simulink model "physical_architecture"  (R2019b)
settings: Solver=VariableStepAuto  StartTime=0.0  StopTime=10.0  RelTol=1e-3
settings Model: Creator=nicol  LastModifiedBy=nicol

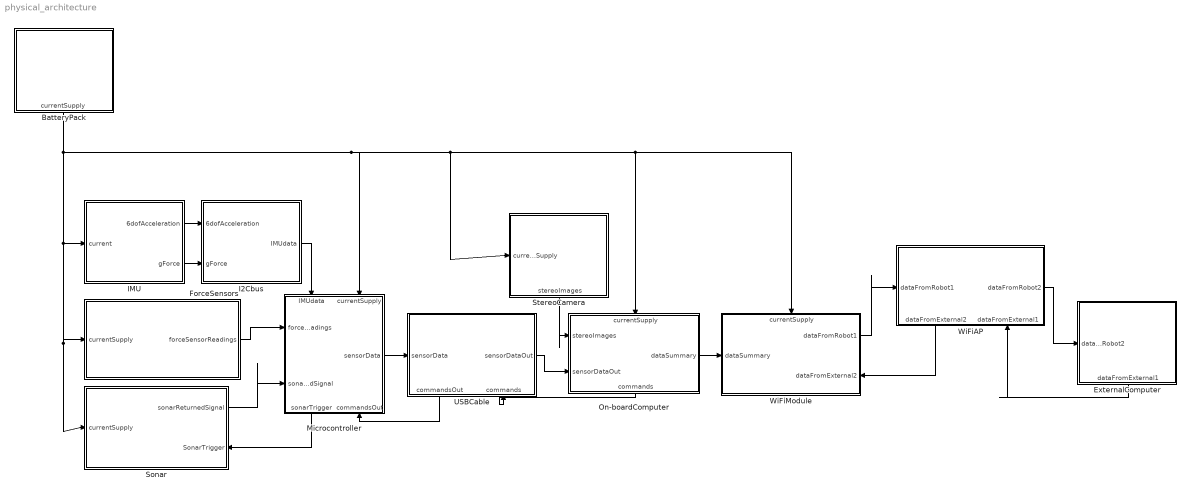
== system physical_architecture ==
  BatteryPack : Subsystem
      settings: PortSchema="{\"entries\":[{\"content\":{\"headerSize\":26,\"margin\":15,\"minimumSpacing\":25,\"sides\":[{\"content\":{\"connectorIds\":[]},\"type\":\"ConnectorPlacement.EquallySpacedRectSide\",\"uuid\":\"1a5b96a6-6b68-4a44-94ba-f4f30127e72c\"},{\"content\":{\"connectorIds\":[],\"side\":\"RIGHT\"},\"type\":\"ConnectorPlacement.EquallySpacedRectSide\",\"uuid\":\"6795999a-37c2-4f74-9b2a-5ff47da3b2b8\"},{\"content\":{\"connectorIds\":[],\"side\":\"TOP\"},\"type\":\"ConnectorPlacement.EquallySpacedRectSide\",\"uuid\":\"71a167ad-2262-404f-8290-656c4c9ef881\"},{\"content\":{\"connectorIds\":[\"Out1\"],\"side\":\"BOTTOM\"},\"type\":\"ConnectorPlacement.EquallySpacedRectSide\",\"uuid\":\"0e7f1ae4-2808-47ff-a788-11b0bf7ea7a5\"}]},\"type\":\"ConnectorPlacement.EquallySpacedConnector\",\"uuid\":\"f8e426a6-4f1d-49ba-8aa9-835f0600076a\"}],\"packageUris\":[\"http://schema.mathworks.com/mf0/Connector/19700101\"],\"version\":\"1.0\"}"
  ExternalComputer : Subsystem
      settings: PortSchema="{\"entries\":[{\"content\":{\"headerSize\":26,\"margin\":15,\"minimumSpacing\":25,\"sides\":[{\"content\":{\"connectorIds\":[\"In1\"]},\"type\":\"ConnectorPlacement.EquallySpacedRectSide\",\"uuid\":\"1a5b96a6-6b68-4a44-94ba-f4f30127e72c\"},{\"content\":{\"connectorIds\":[],\"side\":\"RIGHT\"},\"type\":\"ConnectorPlacement.EquallySpacedRectSide\",\"uuid\":\"6795999a-37c2-4f74-9b2a-5ff47da3b2b8\"},{\"content\":{\"connectorIds\":[],\"side\":\"TOP\"},\"type\":\"ConnectorPlacement.EquallySpacedRectSide\",\"uuid\":\"71a167ad-2262-404f-8290-656c4c9ef881\"},{\"content\":{\"connectorIds\":[\"Out1\"],\"side\":\"BOTTOM\"},\"type\":\"ConnectorPlacement.EquallySpacedRectSide\",\"uuid\":\"2cc7744c-30d7-486d-8de8-8132ed659702\"}]},\"type\":\"ConnectorPlacement.EquallySpacedConnector\",\"uuid\":\"f8e426a6-4f1d-49ba-8aa9-835f0600076a\"}],\"packageUris\":[\"http://schema.mathworks.com/mf0/Connector/19700101\"],\"version\":\"1.0\"}"
  ForceSensors : Subsystem
      settings: PortSchema="{\"entries\":[{\"content\":{\"headerSize\":26,\"margin\":15,\"minimumSpacing\":25,\"sides\":[{\"content\":{\"connectorIds\":[\"In1\"]},\"type\":\"ConnectorPlacement.EquallySpacedRectSide\",\"uuid\":\"1a5b96a6-6b68-4a44-94ba-f4f30127e72c\"},{\"content\":{\"connectorIds\":[\"Out1\"],\"side\":\"RIGHT\"},\"type\":\"ConnectorPlacement.EquallySpacedRectSide\",\"uuid\":\"6795999a-37c2-4f74-9b2a-5ff47da3b2b8\"},{\"content\":{\"connectorIds\":[],\"side\":\"TOP\"},\"type\":\"ConnectorPlacement.EquallySpacedRectSide\",\"uuid\":\"71a167ad-2262-404f-8290-656c4c9ef881\"}]},\"type\":\"ConnectorPlacement.EquallySpacedConnector\",\"uuid\":\"f8e426a6-4f1d-49ba-8aa9-835f0600076a\"}],\"packageUris\":[\"http://schema.mathworks.com/mf0/Connector/19700101\"],\"version\":\"1.0\"}"
  I2Cbus : Subsystem
      settings: PortSchema="{\"entries\":[{\"content\":{\"headerSize\":26,\"margin\":15,\"minimumSpacing\":25,\"sides\":[{\"content\":{\"connectorIds\":[\"In1\",\"In2\"]},\"type\":\"ConnectorPlacement.EquallySpacedRectSide\",\"uuid\":\"1a5b96a6-6b68-4a44-94ba-f4f30127e72c\"},{\"content\":{\"connectorIds\":[\"Out1\"],\"side\":\"RIGHT\"},\"type\":\"ConnectorPlacement.EquallySpacedRectSide\",\"uuid\":\"6795999a-37c2-4f74-9b2a-5ff47da3b2b8\"},{\"content\":{\"connectorIds\":[],\"side\":\"TOP\"},\"type\":\"ConnectorPlacement.EquallySpacedRectSide\",\"uuid\":\"71a167ad-2262-404f-8290-656c4c9ef881\"}]},\"type\":\"ConnectorPlacement.EquallySpacedConnector\",\"uuid\":\"f8e426a6-4f1d-49ba-8aa9-835f0600076a\"}],\"packageUris\":[\"http://schema.mathworks.com/mf0/Connector/19700101\"],\"version\":\"1.0\"}"
  IMU : Subsystem
      settings: PortSchema="{\"entries\":[{\"content\":{\"headerSize\":26,\"margin\":15,\"minimumSpacing\":25,\"sides\":[{\"content\":{\"connectorIds\":[\"In1\"]},\"type\":\"ConnectorPlacement.EquallySpacedRectSide\",\"uuid\":\"1a5b96a6-6b68-4a44-94ba-f4f30127e72c\"},{\"content\":{\"connectorIds\":[\"Out1\",\"Out2\"],\"side\":\"RIGHT\"},\"type\":\"ConnectorPlacement.EquallySpacedRectSide\",\"uuid\":\"6795999a-37c2-4f74-9b2a-5ff47da3b2b8\"},{\"content\":{\"connectorIds\":[],\"side\":\"TOP\"},\"type\":\"ConnectorPlacement.EquallySpacedRectSide\",\"uuid\":\"71a167ad-2262-404f-8290-656c4c9ef881\"}]},\"type\":\"ConnectorPlacement.EquallySpacedConnector\",\"uuid\":\"f8e426a6-4f1d-49ba-8aa9-835f0600076a\"}],\"packageUris\":[\"http://schema.mathworks.com/mf0/Connector/19700101\"],\"version\":\"1.0\"}"
  Microcontroller : Subsystem
      settings: PortSchema="{\"entries\":[{\"content\":{\"headerSize\":26,\"margin\":15,\"minimumSpacing\":25,\"sides\":[{\"content\":{\"connectorIds\":[\"In2\",\"In4\"]},\"type\":\"ConnectorPlacement.EquallySpacedRectSide\",\"uuid\":\"1a5b96a6-6b68-4a44-94ba-f4f30127e72c\"},{\"content\":{\"connectorIds\":[\"Out1\"],\"side\":\"RIGHT\"},\"type\":\"ConnectorPlacement.EquallySpacedRectSide\",\"uuid\":\"6795999a-37c2-4f74-9b2a-5ff47da3b2b8\"},{\"content\":{\"connectorIds\":[\"In5\",\"In3\"],\"side\":\"TOP\"},\"type\":\"ConnectorPlacement.EquallySpacedRectSide\",\"uuid\":\"71a167ad-2262-404f-8290-656c4c9ef881\"},{\"content\":{\"connectorIds\":[\"Out2\",\"In1\"],\"side\":\"BOTTOM\"},\"type\":\"ConnectorPlacement.EquallySpacedRectSide\",\"uuid\":\"845b4600-6435-40f5-ac3b-dfa55e6d602e\"}]},\"type\":\"ConnectorPlacement.EquallySpacedConnector\",\"uuid\":\"f8e426a6-4f1d-49ba-8aa9-835f0600076a\"}],\"packageUris\":[\"http://schema.mathworks.com/mf0/Connector/19700101\"],\"version\":\"1.0\"}"
  On-boardComputer : Subsystem
      settings: PortSchema="{\"entries\":[{\"content\":{\"headerSize\":26,\"margin\":15,\"minimumSpacing\":25,\"sides\":[{\"content\":{\"connectorIds\":[\"In2\",\"In3\"]},\"type\":\"ConnectorPlacement.EquallySpacedRectSide\",\"uuid\":\"1a5b96a6-6b68-4a44-94ba-f4f30127e72c\"},{\"content\":{\"connectorIds\":[\"Out1\"],\"side\":\"RIGHT\"},\"type\":\"ConnectorPlacement.EquallySpacedRectSide\",\"uuid\":\"6795999a-37c2-4f74-9b2a-5ff47da3b2b8\"},{\"content\":{\"connectorIds\":[\"In1\"],\"side\":\"TOP\"},\"type\":\"ConnectorPlacement.EquallySpacedRectSide\",\"uuid\":\"71a167ad-2262-404f-8290-656c4c9ef881\"},{\"content\":{\"connectorIds\":[\"Out2\"],\"side\":\"BOTTOM\"},\"type\":\"ConnectorPlacement.EquallySpacedRectSide\",\"uuid\":\"e904cf2f-4a71-419b-a2b8-63e25171dc86\"}]},\"type\":\"ConnectorPlacement.EquallySpacedConnector\",\"uuid\":\"f8e426a6-4f1d-49ba-8aa9-835f0600076a\"}],\"packageUris\":[\"http://schema.mathworks.com/mf0/Connector/19700101\"],\"version\":\"1.0\"}"
  Sonar : Subsystem
      settings: PortSchema="{\"entries\":[{\"content\":{\"headerSize\":26,\"margin\":15,\"minimumSpacing\":25,\"sides\":[{\"content\":{\"connectorIds\":[\"In1\"]},\"type\":\"ConnectorPlacement.EquallySpacedRectSide\",\"uuid\":\"1a5b96a6-6b68-4a44-94ba-f4f30127e72c\"},{\"content\":{\"connectorIds\":[\"Out1\",\"In2\"],\"side\":\"RIGHT\"},\"type\":\"ConnectorPlacement.EquallySpacedRectSide\",\"uuid\":\"6795999a-37c2-4f74-9b2a-5ff47da3b2b8\"},{\"content\":{\"connectorIds\":[],\"side\":\"TOP\"},\"type\":\"ConnectorPlacement.EquallySpacedRectSide\",\"uuid\":\"71a167ad-2262-404f-8290-656c4c9ef881\"}]},\"type\":\"ConnectorPlacement.EquallySpacedConnector\",\"uuid\":\"f8e426a6-4f1d-49ba-8aa9-835f0600076a\"}],\"packageUris\":[\"http://schema.mathworks.com/mf0/Connector/19700101\"],\"version\":\"1.0\"}"
  StereoCamera : Subsystem
      settings: PortSchema="{\"entries\":[{\"content\":{\"headerSize\":26,\"margin\":15,\"minimumSpacing\":25,\"sides\":[{\"content\":{\"connectorIds\":[\"In1\"]},\"type\":\"ConnectorPlacement.EquallySpacedRectSide\",\"uuid\":\"1a5b96a6-6b68-4a44-94ba-f4f30127e72c\"},{\"content\":{\"connectorIds\":[],\"side\":\"RIGHT\"},\"type\":\"ConnectorPlacement.EquallySpacedRectSide\",\"uuid\":\"6795999a-37c2-4f74-9b2a-5ff47da3b2b8\"},{\"content\":{\"connectorIds\":[],\"side\":\"TOP\"},\"type\":\"ConnectorPlacement.EquallySpacedRectSide\",\"uuid\":\"71a167ad-2262-404f-8290-656c4c9ef881\"},{\"content\":{\"connectorIds\":[\"Out1\"],\"side\":\"BOTTOM\"},\"type\":\"ConnectorPlacement.EquallySpacedRectSide\",\"uuid\":\"983849b7-be9a-4e5c-b816-a95c1f7f6796\"}]},\"type\":\"ConnectorPlacement.EquallySpacedConnector\",\"uuid\":\"f8e426a6-4f1d-49ba-8aa9-835f0600076a\"}],\"packageUris\":[\"http://schema.mathworks.com/mf0/Connector/19700101\"],\"version\":\"1.0\"}"
  USBCable : Subsystem
      settings: PortSchema="{\"entries\":[{\"content\":{\"headerSize\":26,\"margin\":15,\"minimumSpacing\":25,\"sides\":[{\"content\":{\"connectorIds\":[\"In2\"]},\"type\":\"ConnectorPlacement.EquallySpacedRectSide\",\"uuid\":\"1a5b96a6-6b68-4a44-94ba-f4f30127e72c\"},{\"content\":{\"connectorIds\":[\"Out2\"],\"side\":\"RIGHT\"},\"type\":\"ConnectorPlacement.EquallySpacedRectSide\",\"uuid\":\"6795999a-37c2-4f74-9b2a-5ff47da3b2b8\"},{\"content\":{\"connectorIds\":[],\"side\":\"TOP\"},\"type\":\"ConnectorPlacement.EquallySpacedRectSide\",\"uuid\":\"71a167ad-2262-404f-8290-656c4c9ef881\"},{\"content\":{\"connectorIds\":[\"Out1\",\"In1\"],\"side\":\"BOTTOM\"},\"type\":\"ConnectorPlacement.EquallySpacedRectSide\",\"uuid\":\"96aedcb9-6a36-4cb0-8a83-77dcedd4fe91\"}]},\"type\":\"ConnectorPlacement.EquallySpacedConnector\",\"uuid\":\"f8e426a6-4f1d-49ba-8aa9-835f0600076a\"}],\"packageUris\":[\"http://schema.mathworks.com/mf0/Connector/19700101\"],\"version\":\"1.0\"}"
  WiFiAP : Subsystem
      settings: PortSchema="{\"entries\":[{\"content\":{\"headerSize\":26,\"margin\":15,\"minimumSpacing\":25,\"sides\":[{\"content\":{\"connectorIds\":[\"In2\"]},\"type\":\"ConnectorPlacement.EquallySpacedRectSide\",\"uuid\":\"1a5b96a6-6b68-4a44-94ba-f4f30127e72c\"},{\"content\":{\"connectorIds\":[\"Out2\"],\"side\":\"RIGHT\"},\"type\":\"ConnectorPlacement.EquallySpacedRectSide\",\"uuid\":\"6795999a-37c2-4f74-9b2a-5ff47da3b2b8\"},{\"content\":{\"connectorIds\":[],\"side\":\"TOP\"},\"type\":\"ConnectorPlacement.EquallySpacedRectSide\",\"uuid\":\"71a167ad-2262-404f-8290-656c4c9ef881\"},{\"content\":{\"connectorIds\":[\"Out1\",\"In1\"],\"side\":\"BOTTOM\"},\"type\":\"ConnectorPlacement.EquallySpacedRectSide\",\"uuid\":\"aacabda8-2325-475d-956c-e2fb6a2fac11\"}]},\"type\":\"ConnectorPlacement.EquallySpacedConnector\",\"uuid\":\"f8e426a6-4f1d-49ba-8aa9-835f0600076a\"}],\"packageUris\":[\"http://schema.mathworks.com/mf0/Connector/19700101\"],\"version\":\"1.0\"}"
  WiFiModule : Subsystem
      settings: PortSchema="{\"entries\":[{\"content\":{\"headerSize\":26,\"margin\":15,\"minimumSpacing\":25,\"sides\":[{\"content\":{\"connectorIds\":[\"In3\"]},\"type\":\"ConnectorPlacement.EquallySpacedRectSide\",\"uuid\":\"1a5b96a6-6b68-4a44-94ba-f4f30127e72c\"},{\"content\":{\"connectorIds\":[\"Out1\",\"In2\"],\"side\":\"RIGHT\"},\"type\":\"ConnectorPlacement.EquallySpacedRectSide\",\"uuid\":\"6795999a-37c2-4f74-9b2a-5ff47da3b2b8\"},{\"content\":{\"connectorIds\":[\"In1\"],\"side\":\"TOP\"},\"type\":\"ConnectorPlacement.EquallySpacedRectSide\",\"uuid\":\"71a167ad-2262-404f-8290-656c4c9ef881\"}]},\"type\":\"ConnectorPlacement.EquallySpacedConnector\",\"uuid\":\"f8e426a6-4f1d-49ba-8aa9-835f0600076a\"}],\"packageUris\":[\"http://schema.mathworks.com/mf0/Connector/19700101\"],\"version\":\"1.0\"}"
  wires:
  IMU/1(6dofAcceleration) -> I2Cbus/1(6dofAcceleration)
  IMU/2(gForce) -> I2Cbus/2(gForce)
  I2Cbus/1(IMUdata) -> Microcontroller/5(IMUdata)
  ForceSensors/1(forceSensorReadings) -> Microcontroller/2(forceSensorReadings)
  Sonar/1(sonarReturnedSignal) -> Microcontroller/4(sonarReturnedSignal)
  Microcontroller/2(sonarTrigger) -> Sonar/2(SonarTrigger)
  Microcontroller/1(sensorData) -> USBCable/2(sensorData)
  USBCable/2(sensorDataOut) -> On-boardComputer/3(sensorDataOut)
  On-boardComputer/2(commands) -> USBCable/1(commands)
  On-boardComputer/1(dataSummary) -> WiFiModule/3(dataSummary)
  WiFiModule/1(dataFromRobot1) -> WiFiAP/2(dataFromRobot1)
  WiFiAP/2(dataFromRobot2) -> ExternalComputer/1(dataFromRobot2)
  ExternalComputer/1(dataFromExternal1) -> WiFiAP/1(dataFromExternal1)
  WiFiAP/1(dataFromExternal2) -> WiFiModule/2(dataFromExternal2)
  StereoCamera/1(stereoImages) -> On-boardComputer/2(stereoImages)
  BatteryPack/1(currentSupply) -> StereoCamera/1(currentSupply), WiFiModule/1(currentSupply), On-boardComputer/1(currentSupply), Microcontroller/3(currentSupply), Sonar/1(currentSupply), ForceSensors/1(currentSupply), IMU/1(current)
  USBCable/1(commandsOut) -> Microcontroller/1(commandsOut)

== system physical_architecture/BatteryPack ==
  Bus Element Out1 : Outport  PortName=currentSupply

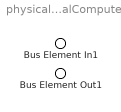
== system physical_architecture/ExternalComputer ==
  Bus Element In1 : Inport  PortName=dataFromRobot2
  Bus Element Out1 : Outport  PortName=dataFromExternal1

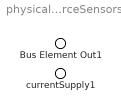
== system physical_architecture/ForceSensors ==
  currentSupply1 : Inport  PortName=currentSupply
  Bus Element Out1 : Outport  PortName=forceSensorReadings

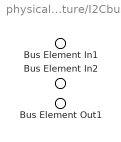
== system physical_architecture/I2Cbus ==
  Bus Element In1 : Inport  PortName=6dofAcceleration
  Bus Element In2 : Inport  Port=2  PortName=gForce
  Bus Element Out1 : Outport  PortName=IMUdata

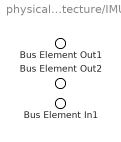
== system physical_architecture/IMU ==
  Bus Element In1 : Inport  PortName=current
  Bus Element Out1 : Outport  PortName=6dofAcceleration
  Bus Element Out2 : Outport  Port=2  PortName=gForce

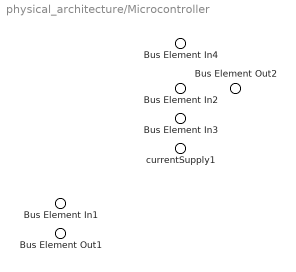
== system physical_architecture/Microcontroller ==
  Bus Element In4 : Inport  PortName=commandsOut
  Bus Element In2 : Inport  Port=2  PortName=forceSensorReadings
  currentSupply1 : Inport  Port=3  PortName=currentSupply
  Bus Element In3 : Inport  Port=4  PortName=sonarReturnedSignal
  Bus Element In1 : Inport  Port=5  PortName=IMUdata
  Bus Element Out2 : Outport  PortName=sensorData
  Bus Element Out1 : Outport  Port=2  PortName=sonarTrigger

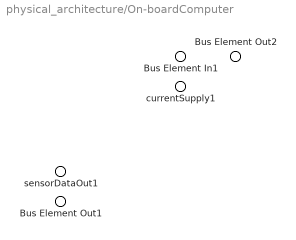
== system physical_architecture/On-boardComputer ==
  currentSupply1 : Inport  PortName=currentSupply
  Bus Element In1 : Inport  Port=2  PortName=stereoImages
  sensorDataOut1 : Inport  Port=3  PortName=sensorDataOut
  Bus Element Out2 : Outport  PortName=dataSummary
  Bus Element Out1 : Outport  Port=2  PortName=commands

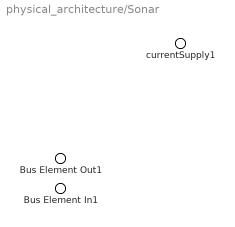
== system physical_architecture/Sonar ==
  currentSupply1 : Inport  PortName=currentSupply
  Bus Element In1 : Inport  Port=2  PortName=SonarTrigger
  Bus Element Out1 : Outport  PortName=sonarReturnedSignal

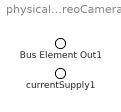
== system physical_architecture/StereoCamera ==
  currentSupply1 : Inport  PortName=currentSupply
  Bus Element Out1 : Outport  PortName=stereoImages

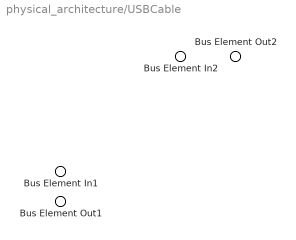
== system physical_architecture/USBCable ==
  Bus Element In2 : Inport  PortName=commands
  Bus Element In1 : Inport  Port=2  PortName=sensorData
  Bus Element Out2 : Outport  PortName=commandsOut
  Bus Element Out1 : Outport  Port=2  PortName=sensorDataOut

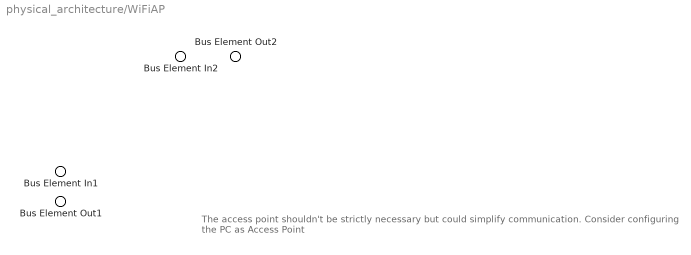
== system physical_architecture/WiFiAP ==
  note: The access point shouldn't be strictly necessary but could simplify communication.
      | Consider configuring the PC as Access Point
  Bus Element In2 : Inport  PortName=dataFromExternal1
  Bus Element In1 : Inport  Port=2  PortName=dataFromRobot1
  Bus Element Out2 : Outport  PortName=dataFromExternal2
  Bus Element Out1 : Outport  Port=2  PortName=dataFromRobot2

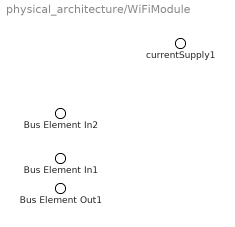
== system physical_architecture/WiFiModule ==
  currentSupply1 : Inport  PortName=currentSupply
  Bus Element In2 : Inport  Port=2  PortName=dataFromExternal2
  Bus Element In1 : Inport  Port=3  PortName=dataSummary
  Bus Element Out1 : Outport  PortName=dataFromRobot1
